simulink model "nauni_fieldtesting"  (R2025b)
settings: Solver=FixedStepDiscrete  StartTime=0.0  StopTime=259200  FixedStep=1  RelTol=1e-3
InitFcn:
  | init_nauni;
  | set_param(bdroot,'StopTime',num2str(StopTime));
undefined symbols (not defined in the file): a, a_soil, DiscIntNeverNeededParam, evap_rate, noise, rain_every_hours, rain_pulse, RH_amp, RH_mean, T_amp, T_mean, Ts, Tsoil_amp, Tsoil_lag_h, Tsoil_mean, VWC_init, VWC_max, VWC_min
libraries: simulink x4
settings Model: Creator=Hunny  LastModifiedBy=Hunny
settings DataIOCC: SaveState=on

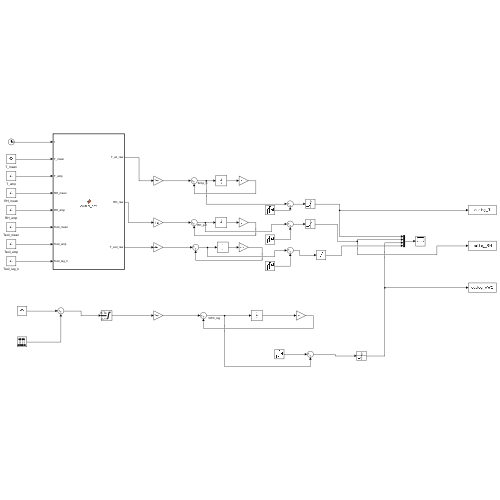
[thumbnail: Simulink's stored preview of the top-level diagram]
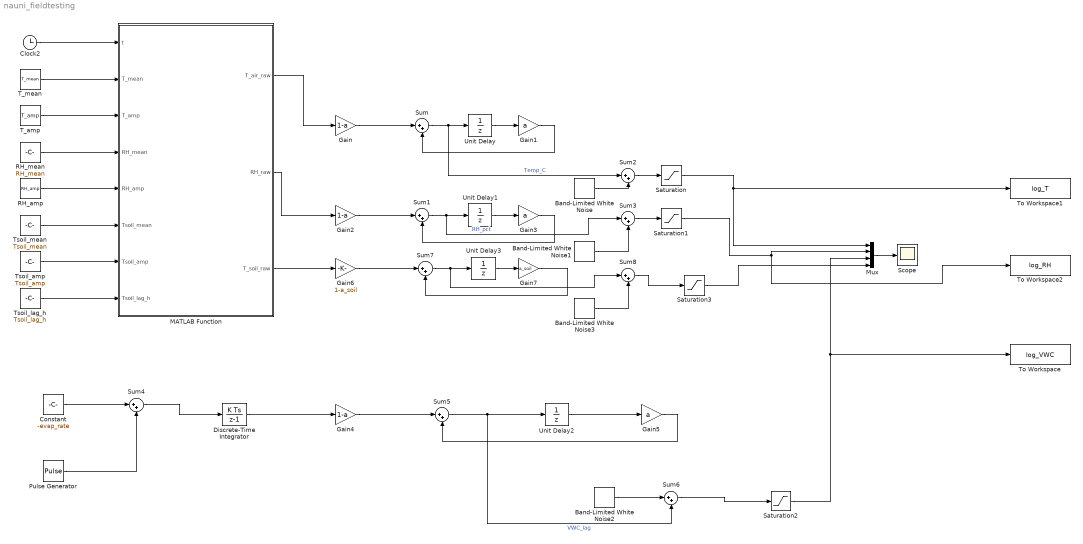
== system nauni_fieldtesting ==
  Band-Limited White Noise : simulink/Sources/Band-Limited White Noise  Cov=noise.T^2  Ts=Ts  seed=[23341]
  Band-Limited White Noise1 : simulink/Sources/Band-Limited White Noise  Cov=noise.RH^2  Ts=Ts  seed=[23341]
  Band-Limited White Noise2 : simulink/Sources/Band-Limited White Noise  Cov=noise.VWC^2,  Ts=Ts  seed=[23341]
  Band-Limited White Noise3 : simulink/Sources/Band-Limited White Noise  Cov=noise.Tsoil^2  Ts=Ts  seed=[23341]
  Clock2 : Clock
  Constant : Constant  Value=-evap_rate  SampleTime=Ts
  Discrete-Time Integrator : DiscreteIntegrator  InitialCondition=VWC_init  SampleTime=Ts  LimitOutput=on  ICPrevOutput=DiscIntNeverNeededParam  ICPrevScaledInput=DiscIntNeverNeededParam
  Gain : Gain  Gain=1-a
  Gain1 : Gain  Gain=a
  Gain2 : Gain  Gain=1-a
  Gain3 : Gain  Gain=a
  Gain4 : Gain  Gain=1-a
  Gain5 : Gain  Gain=a
  Gain6 : Gain  Gain=1-a_soil
  Gain7 : Gain  Gain=a_soil
  MATLAB Function : MATLAB Function  TreatAsAtomicUnit=on
  Mux : Mux
  Pulse Generator : DiscretePulseGenerator  Amplitude=rain_pulse  Period=rain_every_hours*3600  SampleTime=Ts
  RH_amp : Constant  Value=RH_amp
  RH_mean : Constant  Value=RH_mean
  Saturation : Saturate  UpperLimit=50  LowerLimit=-10
  Saturation1 : Saturate  UpperLimit=100  LowerLimit=30
  Saturation2 : Saturate  UpperLimit=VWC_max  LowerLimit=VWC_min
  Saturation3 : Saturate  UpperLimit=40  LowerLimit=0
  Scope : Scope
      settings: ActiveDisplayYMinimum=-60.732309396451413  ActiveDisplayYMaximum=94.217451183925121
  Sum{,1..8} (9 alike) : Sum  Inputs=|++
  T_amp : Constant  Value=T_amp
  T_mean : Constant  Value=T_mean
  To Workspace : ToWorkspace  VariableName=log_VWC  SaveFormat=Structure With Time  SampleTime=Ts
  To Workspace1 : ToWorkspace  VariableName=log_T  SaveFormat=Structure With Time  SampleTime=Ts
  To Workspace2 : ToWorkspace  VariableName=log_RH  SaveFormat=Structure With Time  SampleTime=Ts
  Tsoil_amp : Constant  Value=Tsoil_amp
  Tsoil_lag_h : Constant  Value=Tsoil_lag_h
  Tsoil_mean : Constant  Value=Tsoil_mean
  Unit Delay{,1..3} (4 alike) : UnitDelay  SampleTime=Ts  HasFrameUpgradeWarning=on
  wires:
  Clock2/1 -> MATLAB Function/1(t)
  T_mean/1 -> MATLAB Function/2(T_mean)
  T_amp/1 -> MATLAB Function/3(T_amp)
  RH_mean/1 -> MATLAB Function/4(RH_mean)
  RH_amp/1 -> MATLAB Function/5(RH_amp)
  MATLAB Function/1(T_air_raw) -> Gain/1
  Gain/1 -> Sum/1
  Sum/1 -> Sum2/1, Unit Delay/1  "Temp_C"
  MATLAB Function/2(RH_raw) -> Gain2/1
  Gain2/1 -> Sum1/1
  Sum1/1 -> Sum3/1, Unit Delay1/1  "RH_pct"
  Unit Delay/1 -> Gain1/1
  Gain1/1 -> Sum/2
  Unit Delay1/1 -> Gain3/1
  Gain3/1 -> Sum1/2
  Band-Limited White Noise/1 -> Sum2/2
  Sum2/1 -> Saturation/1
  Band-Limited White Noise1/1 -> Sum3/2
  Sum3/1 -> Saturation1/1
  Constant/1 -> Sum4/1
  Pulse Generator/1 -> Sum4/2
  Sum4/1 -> Discrete-Time Integrator/1
  Sum5/1 -> Sum6/2, Unit Delay2/1  "VWC_lag"
  Unit Delay2/1 -> Gain5/1
  Gain5/1 -> Sum5/2
  Band-Limited White Noise2/1 -> Sum6/1
  Sum6/1 -> Saturation2/1
  Saturation/1 -> Mux/1, To Workspace1/1
  Mux/1 -> Scope/1
  Saturation1/1 -> To Workspace2/1, Mux/2
  Saturation2/1 -> Mux/3, To Workspace/1
  Discrete-Time Integrator/1 -> Gain4/1
  Gain4/1 -> Sum5/1
  Tsoil_mean/1 -> MATLAB Function/6(Tsoil_mean)
  Tsoil_amp/1 -> MATLAB Function/7(Tsoil_amp)
  Tsoil_lag_h/1 -> MATLAB Function/8(Tsoil_lag_h)
  Gain6/1 -> Sum7/1
  Sum7/1 -> Sum8/1, Unit Delay3/1
  Unit Delay3/1 -> Gain7/1
  Gain7/1 -> Sum7/2
  Band-Limited White Noise3/1 -> Sum8/2
  Sum8/1 -> Saturation3/1
  MATLAB Function/3(T_soil_raw) -> Gain6/1
  Saturation3/1 -> Mux/4

== matlab function nauni_fieldtesting/MATLAB Function ==
  data: t input; T_air_raw output; T_mean input; T_amp input; RH_mean input; RH_amp input; RH_raw output; Tsoil_mean input; Tsoil_amp input; Tsoil_lag_h input; T_soil_raw output
function [T_air_raw, RH_raw, T_soil_raw] = diurnal_env( ...
    t, T_mean, T_amp, RH_mean, RH_amp, ...
    Tsoil_mean, Tsoil_amp, Tsoil_lag_h)

hr = mod(t/3600, 24);

% Air temperature
T_air_raw = T_mean + T_amp * sin(2*pi*(hr - 5)/24);

% Relative humidity
RH_raw = RH_mean + RH_amp * sin(2*pi*(hr + 7)/24);

% Soil temperature: delayed & smaller swing
T_soil_raw = Tsoil_mean + Tsoil_amp * ...
             sin(2*pi*(hr - 5 - Tsoil_lag_h)/24);
end
